simulink model "lqr_lineal_model"  (R2018a)
settings: Solver=VariableStepAuto  StartTime=0.0  StopTime=10.0  RelTol=1e-3
undefined symbols (not defined in the file): K, sys
settings Model: Creator=Mrcs641  LastModifiedBy=Mrcs641

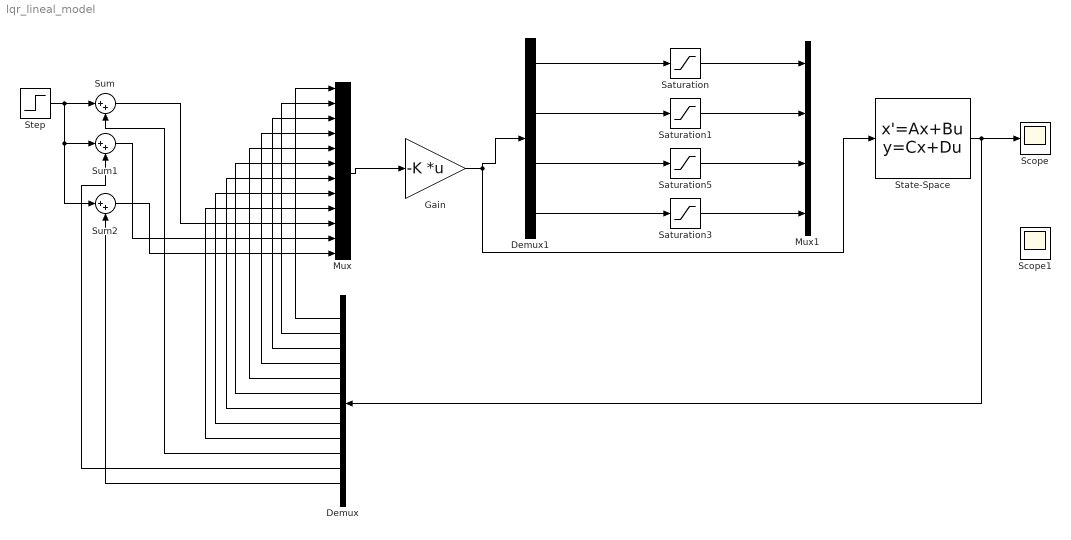
== system lqr_lineal_model ==
  Demux : Demux  Outputs=12
  Demux1 : Demux
  Gain : Gain  Gain=-K  Multiplication=Matrix(K*u)
  Mux : Mux  Inputs=12
  Mux1 : Mux
  Saturation : Saturate  UpperLimit=20  LowerLimit=0  LinearizeAsGain=off  ZeroCross=off
  Saturation1 : Saturate  UpperLimit=10  LowerLimit=-10  LinearizeAsGain=off  ZeroCross=off
  Saturation3 : Saturate  UpperLimit=10  LowerLimit=-10  LinearizeAsGain=off  ZeroCross=off
  Saturation5 : Saturate  UpperLimit=10  LowerLimit=-10  LinearizeAsGain=off  ZeroCross=off
  Scope : Scope
  Scope1 : Scope
  State-Space : StateSpace  A=sys.A  B=sys.B  C=sys.C  D=sys.D  InitialCondition=zeros(1,12)
  Step : Step  Time=2  After=-1  SampleTime=0
  Sum : Sum  Inputs=|++
  Sum1 : Sum  Inputs=|++
  Sum2 : Sum  Inputs=|++
  wires:
  State-Space/1 -> Demux/1, Scope/1
  Step/1 -> Sum2/1, Sum1/1, Sum/1
  Mux/1 -> Gain/1
  Saturation3/1 -> Mux1/4
  Saturation5/1 -> Mux1/3
  Saturation/1 -> Mux1/1
  Saturation1/1 -> Mux1/2
  Gain/1 -> Demux1/1, State-Space/1
  Demux1/1 -> Saturation/1
  Demux1/2 -> Saturation1/1
  Demux1/3 -> Saturation5/1
  Demux1/4 -> Saturation3/1
  Demux/1 -> Mux/1
  Demux/2 -> Mux/2
  Demux/3 -> Mux/3
  Demux/4 -> Mux/4
  Demux/5 -> Mux/5
  Demux/6 -> Mux/6
  Demux/7 -> Mux/7
  Demux/8 -> Mux/8
  Demux/9 -> Mux/9
  Demux/12 -> Sum2/2
  Sum2/1 -> Mux/12
  Demux/11 -> Sum1/2
  Sum1/1 -> Mux/11
  Demux/10 -> Sum/2
  Sum/1 -> Mux/10
